simulink model "SatDynamics"  (R2017a)
settings: Solver=VariableStepAuto  StartTime=0.0  StopTime=200  RelTol=1e-3
undefined symbols (not defined in the file): DiscIntNeverNeededParam
libraries: vrlib x6, simulink x6, aerolibutil x3, shared6dof x2, aerolibanim x1
settings Model: Creator=Simon  LastModifiedBy=Simon

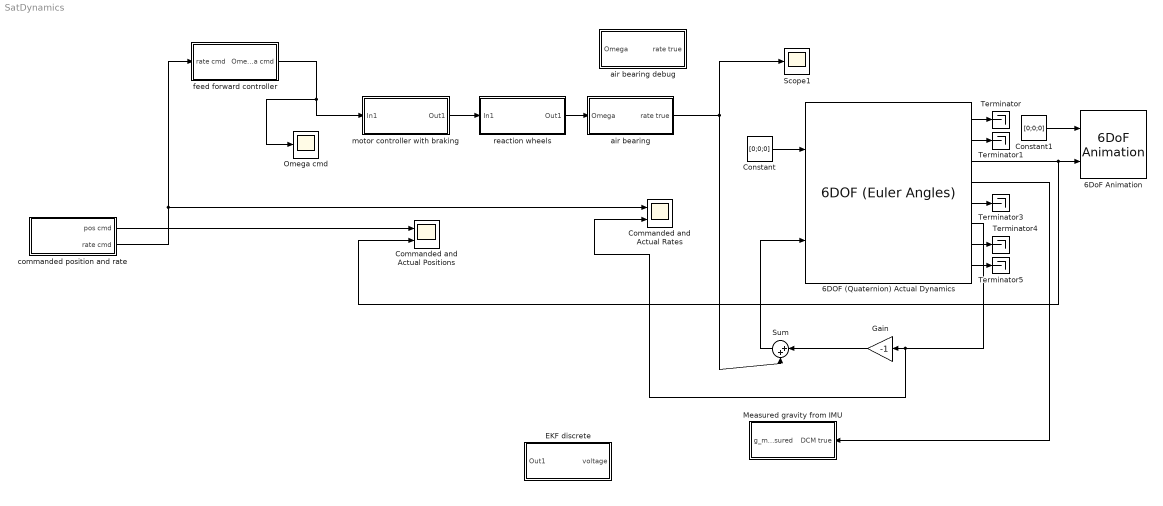
== system SatDynamics ==
  6DOF (Quaternion) Actual Dynamics : shared6dof/6DOF (Euler Angles)  units=Metric (MKS)  mtype=Fixed  rep=Quaternion  xme_0=[0 0 0]  Vm_0=[0 0 0]  eul_0=[0 0 0]  pm_0=[0 0 0]  mass_0=1.0  mass_e=0.5  mass_f=2.0  inertia=0.01*eye(3)  inertia_e=eye(3)  inertia_f=2*eye(3)  k_quat=1.0  vre_flag=on  abi_flag=off
  6DoF Animation : aerolibanim/6DoF Animation  u1=[0 4000 -2000 2000 -5000 -3000]  u2=0.1  u3=1.0  u4=[4000 0 -5000]  u5=Fly alongside  u6=[0 10 0]  u7=10  u8=on
      settings: SourceProductName=Aerospace Blockset
  Commanded and Actual Positions : Scope  NumInputPorts=2
  Commanded and Actual Rates : Scope  NumInputPorts=2
  Constant : Constant  Value=[0;0;0]
  Constant1 : Constant  Value=[0;0;0]
  EKF discrete : Subsystem
  Gain : Gain  Gain=-1
  Measured gravity from IMU : Subsystem
  Omega cmd : Scope
  Scope1 : Scope
  Sum : Sum  Inputs=|++
  Terminator{,1,3..5} (5 alike) : Terminator
  "air bearing " : Subsystem
  air bearing debug : Subsystem
  commanded position and rate : Subsystem
  feed forward controller : Subsystem
  motor controller with braking : Subsystem
  reaction wheels : Subsystem
  wires:
  "air bearing "/1(rate true) -> Sum/2, Scope1/1
  6DOF (Quaternion) Actual Dynamics/6 -> Commanded and Actual Rates/2, Gain/1
  Gain/1 -> Sum/1
  Sum/1 -> 6DOF (Quaternion) Actual Dynamics/2
  6DOF (Quaternion) Actual Dynamics/3 -> Commanded and Actual Positions/2, 6DoF Animation/2
  reaction wheels/1(Out1) -> "air bearing "/1(Omega)
  motor controller with braking/1(Out1) -> reaction wheels/1(In1)
  feed forward controller/1(Omega cmd) -> Omega cmd/1, motor controller with braking/1(In1)
  Constant/1 -> 6DOF (Quaternion) Actual Dynamics/1
  Constant1/1 -> 6DoF Animation/1
  6DOF (Quaternion) Actual Dynamics/1 -> Terminator/1
  6DOF (Quaternion) Actual Dynamics/2 -> Terminator1/1
  6DOF (Quaternion) Actual Dynamics/4 -> Measured gravity from IMU/1(DCM true)
  6DOF (Quaternion) Actual Dynamics/5 -> Terminator3/1
  6DOF (Quaternion) Actual Dynamics/7 -> Terminator4/1
  6DOF (Quaternion) Actual Dynamics/8 -> Terminator5/1
  commanded position and rate/2(rate cmd) -> Commanded and Actual Rates/1, feed forward controller/1(rate cmd)
  commanded position and rate/1(pos cmd) -> Commanded and Actual Positions/1

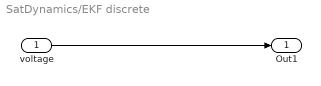
== system SatDynamics/EKF discrete ==
  voltage : Inport
  Out1 : Outport
  wires:
  voltage/1 -> Out1/1

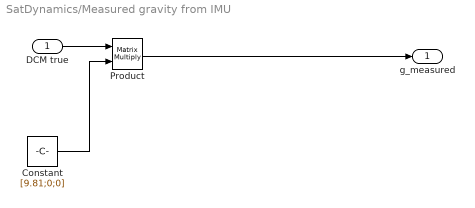
== system SatDynamics/Measured gravity from IMU ==
  DCM true : Inport
  Constant : Constant  Value=[9.81;0;0]
  Product : Product  Multiplication=Matrix(*)
  g_measured : Outport
  wires:
  DCM true/1 -> Product/1
  Constant/1 -> Product/2
  Product/1 -> g_measured/1

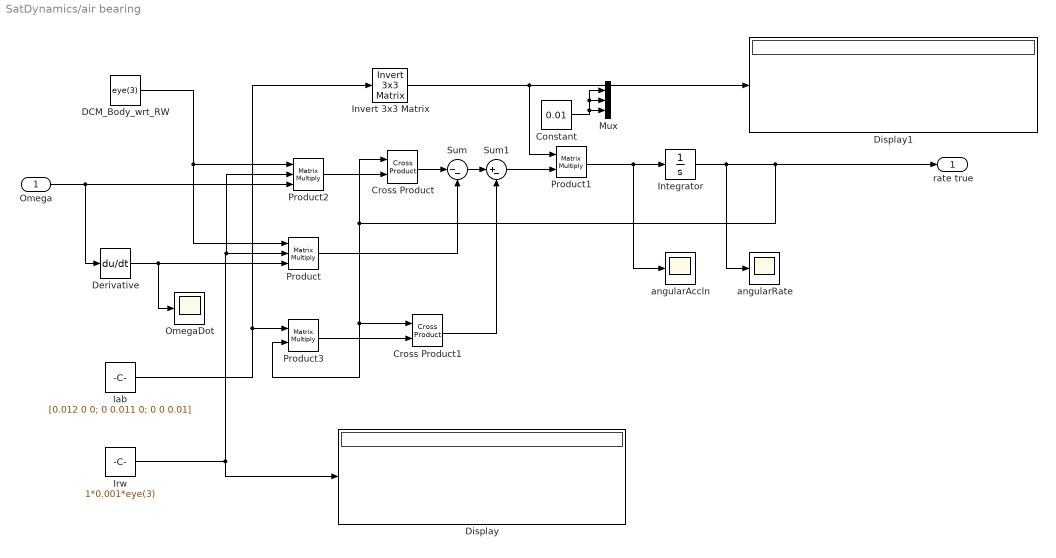
== system SatDynamics/air bearing  ==
  Omega : Inport
  Constant : Constant  Value=0.01
  Cross Product : vrlib/Utilities/Cross Product
      settings: SourceProductBaseCode=VR
  Cross Product1 : vrlib/Utilities/Cross Product
      settings: SourceProductBaseCode=VR
  DCM_Body_wrt_RW : Constant  Value=eye(3)
  Derivative : Derivative  CoefficientInTFapproximation=1
  Display : Display
  Display1 : Display
  Iab : Constant  Value=[0.012 0 0; 0 0.011 0; 0 0 0.01]
  Integrator : Integrator
  Invert 3x3 Matrix : aerolibutil/Invert  3x3 Matrix
  Irw : Constant  Value=1*0.001*eye(3)
  Mux : Mux  Inputs=3
  OmegaDot : Scope
  Product : Product  Inputs=3  Multiplication=Matrix(*)
  Product1 : Product  Multiplication=Matrix(*)
  Product2 : Product  Inputs=3  Multiplication=Matrix(*)
  Product3 : Product  Multiplication=Matrix(*)
  Sum : Sum  Inputs=|--
  Sum1 : Sum  Inputs=|+-
  angularAccln : Scope
  angularRate : Scope
  rate true : Outport
  wires:
  Iab/1 -> Product3/1, Invert 3x3 Matrix/1
  Derivative/1 -> Product/3, OmegaDot/1
  DCM_Body_wrt_RW/1 -> Product2/1, Product/1
  Irw/1 -> Product2/2, Product/2, Display/1
  Product/1 -> Sum/2
  Integrator/1 -> angularRate/1, rate true/1, Cross Product/1, Cross Product1/1, Product3/2
  Omega/1 -> Product2/3, Derivative/1
  Cross Product/1 -> Sum/1
  Sum/1 -> Sum1/1
  Invert 3x3 Matrix/1 -> Product1/1, Display1/1
  Sum1/1 -> Product1/2
  Product3/1 -> Cross Product1/2
  Cross Product1/1 -> Sum1/2
  Product2/1 -> Cross Product/2
  Product1/1 -> Integrator/1, angularAccln/1
  Constant/1 -> Mux/3, Mux/2, Mux/1

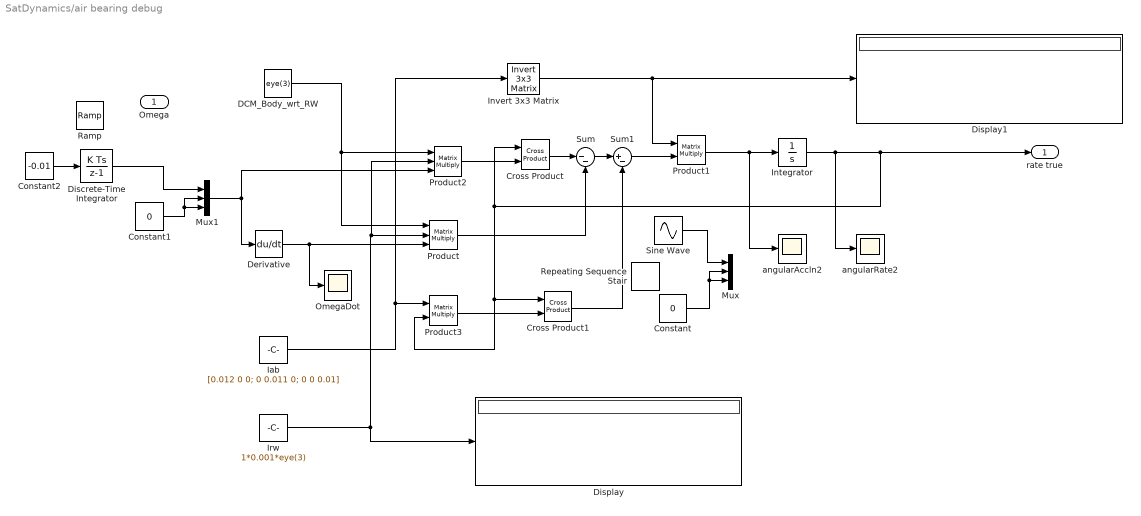
== system SatDynamics/air bearing debug ==
  Omega : Inport
  Constant : Constant  Value=0
  Constant1 : Constant  Value=0
  Constant2 : Constant  Value=-0.01
  Cross Product : vrlib/Utilities/Cross Product
      settings: SourceProductBaseCode=VR
  Cross Product1 : vrlib/Utilities/Cross Product
      settings: SourceProductBaseCode=VR
  DCM_Body_wrt_RW : Constant  Value=eye(3)
  Derivative : Derivative  CoefficientInTFapproximation=1
  Discrete-Time Integrator : DiscreteIntegrator  InitialConditionSetting=State (most efficient)  SampleTime=0.1  ICPrevOutput=DiscIntNeverNeededParam  ICPrevScaledInput=DiscIntNeverNeededParam
  Display : Display
  Display1 : Display
  Iab : Constant  Value=[0.012 0 0; 0 0.011 0; 0 0 0.01]
  Integrator : Integrator
  Invert 3x3 Matrix : aerolibutil/Invert  3x3 Matrix
  Irw : Constant  Value=1*0.001*eye(3)
  Mux : Mux  Inputs=3
  Mux1 : Mux  Inputs=3
  OmegaDot : Scope
  Product : Product  Inputs=3  Multiplication=Matrix(*)
  Product1 : Product  Multiplication=Matrix(*)
  Product2 : Product  Inputs=3  Multiplication=Matrix(*)
  Product3 : Product  Multiplication=Matrix(*)
  Ramp : simulink/Sources/Ramp  slope=-0.01  start=0  X0=0
  Repeating Sequence Stair : simulink/Sources/Repeating Sequence Stair  OutValues=[.01].'  tsamp=1  OutMin=[]  OutMax=[]  OutDataTypeStr=double  OutputDataTypeScalingMode=double  OutDataType=fixdt(0,8)  ConRadixGroup=Best Precision: Vector-wise  OutScaling=2^-12
  Sine Wave : Sin  Amplitude=0.01  Frequency=.1  Phase=pi/2  SampleTime=0
  Sum : Sum  Inputs=|--
  Sum1 : Sum  Inputs=|+-
  angularAccln2 : Scope
  angularRate2 : Scope
  rate true : Outport
  wires:
  Iab/1 -> Product3/1, Invert 3x3 Matrix/1
  Derivative/1 -> Product/3, OmegaDot/1
  DCM_Body_wrt_RW/1 -> Product2/1, Product/1
  Irw/1 -> Product2/2, Product/2, Display/1
  Product/1 -> Sum/2
  Integrator/1 -> angularRate2/1, rate true/1, Cross Product/1, Cross Product1/1, Product3/2
  Mux1/1 -> Product2/3, Derivative/1
  Cross Product/1 -> Sum/1
  Sum/1 -> Sum1/1
  Invert 3x3 Matrix/1 -> Product1/1, Display1/1
  Sum1/1 -> Product1/2
  Product3/1 -> Cross Product1/2
  Cross Product1/1 -> Sum1/2
  Product2/1 -> Cross Product/2
  Product1/1 -> Integrator/1, angularAccln2/1
  Sine Wave/1 -> Mux/1
  Constant/1 -> Mux/3, Mux/2
  Discrete-Time Integrator/1 -> Mux1/1
  Constant1/1 -> Mux1/3, Mux1/2
  Constant2/1 -> Discrete-Time Integrator/1

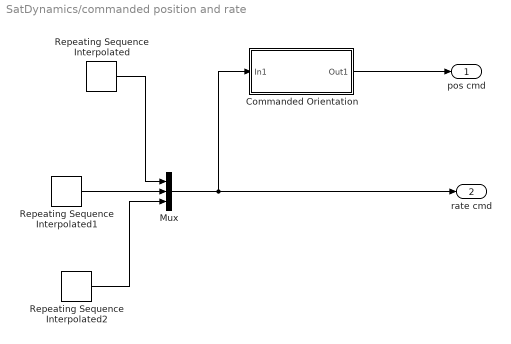
== system SatDynamics/commanded position and rate ==
  Commanded Orientation : Subsystem
  Mux : Mux  Inputs=3
  Repeating Sequence Interpolated : simulink/Sources/Repeating Sequence Interpolated  OutValues=[0 0.2 0 0.1 0]  TimeValues=[0 10 50 60 100].'  LookUpMeth=Interpolation-Use End Values  tsamp=0.01  OutMin=[]  OutMax=[]  OutDataTypeStr=double  OutputDataTypeScalingMode=double  OutDataType=fixdt(0,8)  OutScaling=2^-10
  Repeating Sequence Interpolated1 : simulink/Sources/Repeating Sequence Interpolated  OutValues=[0 -0.1 0 -0.2 0]  TimeValues=[0 10 50 60 100].'  LookUpMeth=Interpolation-Use End Values  tsamp=0.01  OutMin=[]  OutMax=[]  OutDataTypeStr=double  OutputDataTypeScalingMode=double  OutDataType=fixdt(0,8)  OutScaling=2^-10
  Repeating Sequence Interpolated2 : simulink/Sources/Repeating Sequence Interpolated  OutValues=[0 0.15 0 -0.15 0]  TimeValues=[0 10 50 60 100].'  LookUpMeth=Interpolation-Use End Values  tsamp=0.01  OutMin=[]  OutMax=[]  OutDataTypeStr=double  OutputDataTypeScalingMode=double  OutDataType=fixdt(0,8)  OutScaling=2^-10
  pos cmd : Outport
  rate cmd : Outport  Port=2
  wires:
  Mux/1 -> Commanded Orientation/1(In1), rate cmd/1
  Repeating Sequence Interpolated1/1 -> Mux/2
  Repeating Sequence Interpolated/1 -> Mux/1
  Repeating Sequence Interpolated2/1 -> Mux/3
  Commanded Orientation/1(Out1) -> pos cmd/1

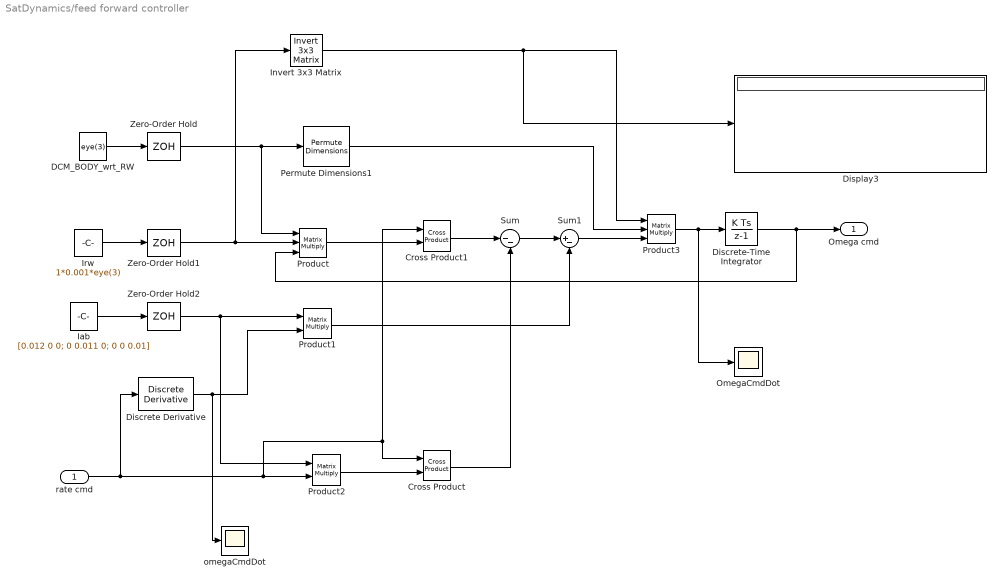
== system SatDynamics/feed forward controller ==
  rate cmd : Inport
  Cross Product : vrlib/Utilities/Cross Product
      settings: SourceProductBaseCode=VR
  Cross Product1 : vrlib/Utilities/Cross Product
      settings: SourceProductBaseCode=VR
  DCM_BODY_wrt_RW : Constant  Value=eye(3)
  Discrete Derivative : simulink/Discrete/Discrete Derivative  gainval=1  ICPrevScaledInput=0.0  OutMin=[]  OutMax=[]  OutDataType=fixdt(1, 16)  OutScaling=2^-10  DoSatur=off
  Discrete-Time Integrator : DiscreteIntegrator  gainval=1  InitialConditionSetting=State (most efficient)  SampleTime=-1  ICPrevOutput=DiscIntNeverNeededParam  ICPrevScaledInput=DiscIntNeverNeededParam
  Display3 : Display
  Iab : Constant  Value=[0.012 0 0; 0 0.011 0; 0 0 0.01]
  Invert 3x3 Matrix : aerolibutil/Invert  3x3 Matrix
  Irw : Constant  Value=1*0.001*eye(3)
  OmegaCmdDot : Scope
  Permute Dimensions1 : PermuteDimensions  Order=[2 1]
  Product : Product  Inputs=3  Multiplication=Matrix(*)
  Product1 : Product  Multiplication=Matrix(*)
  Product2 : Product  Multiplication=Matrix(*)
  Product3 : Product  Inputs=3  Multiplication=Matrix(*)
  Sum : Sum  Inputs=|--
  Sum1 : Sum  Inputs=|+-
  Zero-Order Hold : ZeroOrderHold  SampleTime=-1
  Zero-Order Hold1 : ZeroOrderHold  SampleTime=-1
  Zero-Order Hold2 : ZeroOrderHold  SampleTime=-1
  omegaCmdDot : Scope
  Omega cmd : Outport
  wires:
  rate cmd/1 -> Cross Product/1, Cross Product1/1, Product2/2, Discrete Derivative/1
  DCM_BODY_wrt_RW/1 -> Zero-Order Hold/1
  Irw/1 -> Zero-Order Hold1/1
  Iab/1 -> Zero-Order Hold2/1
  Zero-Order Hold/1 -> Product/1, Permute Dimensions1/1
  Zero-Order Hold1/1 -> Product/2, Invert 3x3 Matrix/1
  Zero-Order Hold2/1 -> Product2/1, Product1/1
  Discrete Derivative/1 -> omegaCmdDot/1, Product1/2
  Product2/1 -> Cross Product/2
  Product/1 -> Cross Product1/2
  Cross Product1/1 -> Sum/1
  Sum/1 -> Sum1/1
  Sum1/1 -> Product3/3
  Invert 3x3 Matrix/1 -> Display3/1, Product3/1
  Permute Dimensions1/1 -> Product3/2
  Product3/1 -> OmegaCmdDot/1, Discrete-Time Integrator/1
  Discrete-Time Integrator/1 -> Product/3, Omega cmd/1
  Cross Product/1 -> Sum/2
  Product1/1 -> Sum1/2

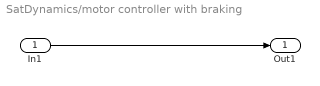
== system SatDynamics/motor controller with braking ==
  In1 : Inport
  Out1 : Outport
  wires:
  In1/1 -> Out1/1

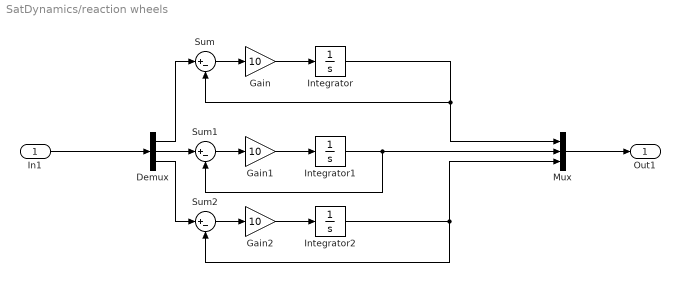
== system SatDynamics/reaction wheels ==
  In1 : Inport
  Demux : Demux  Outputs=3
  Gain : Gain  Gain=10
  Gain1 : Gain  Gain=10
  Gain2 : Gain  Gain=10
  Integrator : Integrator
  Integrator1 : Integrator
  Integrator2 : Integrator
  Mux : Mux  Inputs=3
  Sum : Sum  Inputs=|+-
  Sum1 : Sum  Inputs=|+-
  Sum2 : Sum  Inputs=|+-
  Out1 : Outport
  wires:
  Demux/1 -> Sum/1
  In1/1 -> Demux/1
  Integrator/1 -> Sum/2, Mux/1
  Sum/1 -> Gain/1
  Mux/1 -> Out1/1
  Gain/1 -> Integrator/1
  Demux/2 -> Sum1/1
  Gain1/1 -> Integrator1/1
  Sum1/1 -> Gain1/1
  Integrator1/1 -> Sum1/2, Mux/2
  Integrator2/1 -> Mux/3, Sum2/2
  Sum2/1 -> Gain2/1
  Demux/3 -> Sum2/1
  Gain2/1 -> Integrator2/1

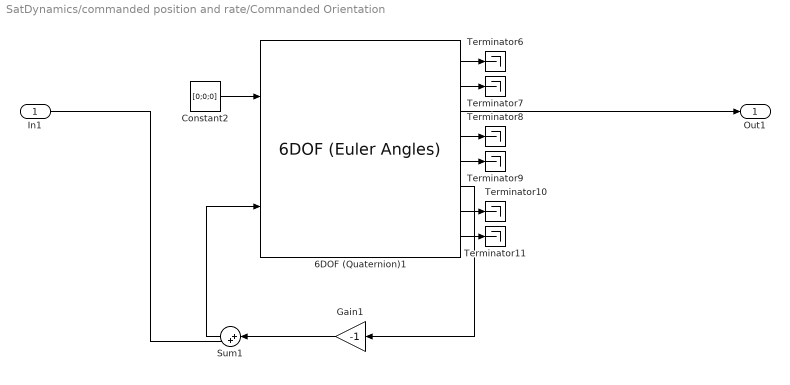
== system SatDynamics/commanded position and rate/Commanded Orientation ==
  In1 : Inport
  6DOF (Quaternion)1 : shared6dof/6DOF (Euler Angles)  units=Metric (MKS)  mtype=Fixed  rep=Quaternion  xme_0=[0 0 0]  Vm_0=[0 0 0]  eul_0=[0 0 0]  pm_0=[0 0 0]  mass_0=1.0  mass_e=0.5  mass_f=2.0  inertia=0.01*eye(3)  inertia_e=eye(3)  inertia_f=2*eye(3)  k_quat=1.0  vre_flag=on  abi_flag=off
  Constant2 : Constant  Value=[0;0;0]
  Gain1 : Gain  Gain=-1
  Sum1 : Sum  Inputs=|++
  Terminator{6..11} (6 alike) : Terminator
  Out1 : Outport
  wires:
  6DOF (Quaternion)1/3 -> Out1/1
  Sum1/1 -> 6DOF (Quaternion)1/2
  6DOF (Quaternion)1/6 -> Gain1/1
  6DOF (Quaternion)1/4 -> Terminator8/1
  6DOF (Quaternion)1/5 -> Terminator9/1
  6DOF (Quaternion)1/2 -> Terminator7/1
  In1/1 -> Sum1/2
  6DOF (Quaternion)1/7 -> Terminator10/1
  Constant2/1 -> 6DOF (Quaternion)1/1
  6DOF (Quaternion)1/8 -> Terminator11/1
  6DOF (Quaternion)1/1 -> Terminator6/1
  Gain1/1 -> Sum1/1
